simulink model "Channelizer_kernel"  (R2024a)
settings: Solver=VariableStepAuto  StartTime=0.0  StopTime=inf  RelTol=1e-3
InitFcn:
  | init
  | init_kernel
values from neighbouring files (symbols this model uses):
  N = 2*1024    (= 2048)    [hil.m]    (also in init.m = 256)
undefined symbols (not defined in the file or in its folder): ch0, ch1, ch10, ch11, ch12, ch13, ch14, ch15, ch2, ch3, ch4, ch5, ch6, ch7, ch8, ch9, S, vsva2197, xcvc1902
libraries: aieBasic x56, aieUtilities x39, hlsBasic x3, dspindex x2, vmcUtilities x1, commchan3 x1, commrflib2 x1, commfilt2 x1, commrandsrc3 x1, commdigbbndam3 x1
(part 1 of 3)
settings Model: Creator=robg  LastModifiedBy=robg
settings DataIOCC: SaveFormat=Array  SaveOutput=off  SignalLogging=off  DSMLogging=off  SaveTime=off
settings OptimizationCC: ReuseModelBlockBuffer=off
settings DebuggingCC: UnconnectedInputMsg=warning  UnconnectedOutputMsg=warning  UnconnectedLineMsg=warning
settings ModelReferenceCC: EnableRefExpFcnMdlSchedulingChecks=on
settings RTWCC: GPUComputeCapability=3.5  DLArmComputeVersion=19.05

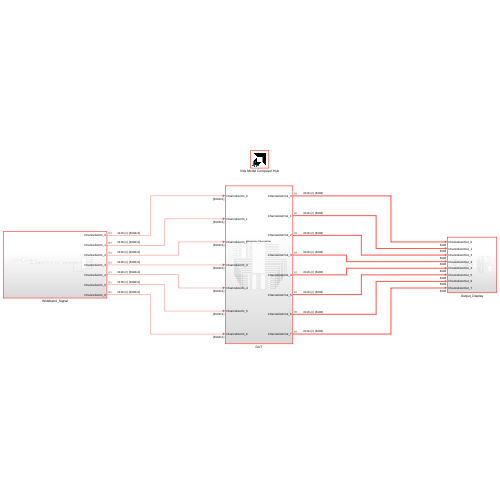
[thumbnail: Simulink's stored preview of the top-level diagram]
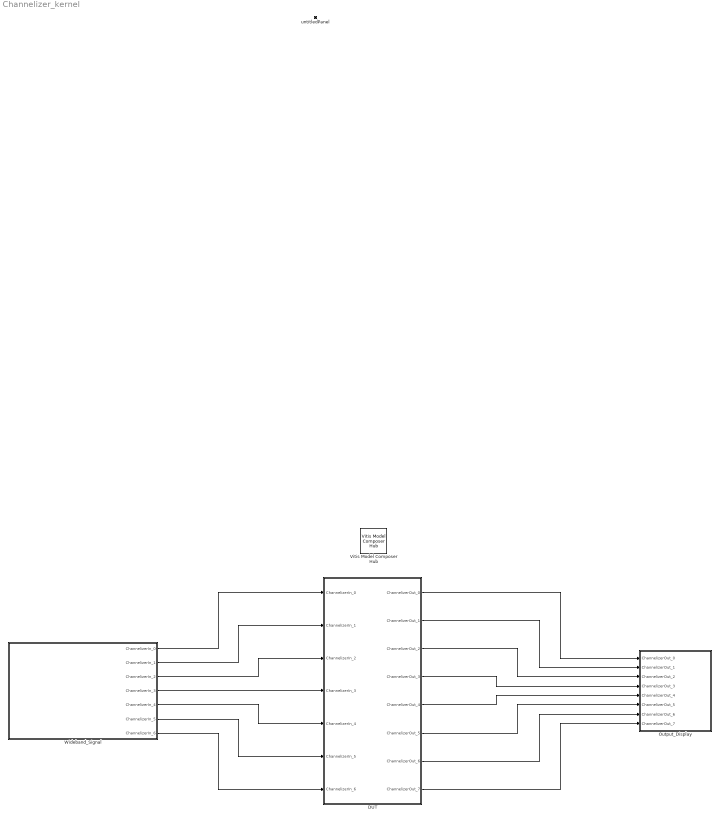
== system Channelizer_kernel ==
  DUT : Subsystem
  Output_Display : Subsystem
  Vitis Model Composer Hub : vmcUtilities/Vitis Model Composer Hub  Tag=genX  CodeGeneration=off  SubsystemName=DUT  DUTSubsystemName=DUT  CompilationType=HWCompilation  SubsystemType=DUTNode  TargetDirectory=./code_hil  exportDesign=off  analyzeDesign=off  validateDesignOnHw=on  ExportType=HW Code  IpVendor=xilinx.com  IpLibrary=hls  IpName=m16_ssr8_permute_fb_o_wrapper  IpVersion=1.0  IpHWLanguage=Verilog  AieCompilerOptions={}  AieSimulatorOptions={}  CreateTestbench=off  TestbenchStackSize=10  RunRtlSim=off  RunCSim=off  RunAieSim=on  AieSimTimeout=50000  RunAieSimProfiling=off  LaunchVitisAnalyzer=off  PlotOutput=off  RunX86Sim=off  X86SimTimeout=10  GenHwImage=off  GenLibadfXo=off  GenHwValidationCode=off  PlatformType=Specify Platform  Platform=/proj/xbuilds/SWIP/2024.1_0306_2227/installs/lin64/Vitis/2024.1/base_platforms/xilinx_vck190_base_202410_1/xilinx_vck190_base_202410_1.xpfm  HwSystemType=Baremetal  HwValidationTarget=hw  ProjDevice=Versal VCK190 Evaluation Platform (xcvc1902-vsva2197-2MP-e-S)  ProjDevicePart=xcvc1902-vsva2197-2MP-e-S  AIEType=AIE  SamplePeriod=-1  ClockFrequency=200  DataPathParallelism=1  xilinxfamily=versalaicore  part=xcvc1902  speed=-2MP-e-S  package=vsva2197  directory=./netlist  testbench=off  incr_netlist=off  synthesis_tool=Vivado  clock_wrapper=Clock Enables  dbl_ovrd=According to Block Masks  dcm_input_clock_period=10  sysclk_period=10  simulink_period=1  eval_field=0  IPInfoJsonString="{\"HLSKernel\":[{\"SubsystemName\":\"m16_ssr8_cyclic_shift_wrapper\",\"IPName\":\"m16_ssr8_cyclic_shift_wrapper\",\"IPLibrary\":\"hls\",\"IPVendor\":\"xilinx.com\",\"IPVersion\":\"1.0\",\"FpgaClockFreq\":\"200\",\"TargetDirectory\":\"./code_hil\",\"SubsystemDir\":\"./code_hil/ip/m16_ssr8_cyclic_shift_wrapper\"},{\"SubsystemName\":\"m16_ssr8_permute_fb_i_wrapper\",\"IPName\":\"m16_ssr8_permute_fb_i_wrapper\",\"IPLibrary\":\"hls\",\"IPVendor\":\"xilinx.com\",\"IPVersion\":\"1.0\",\"FpgaClockFreq\":\"200\",\"TargetDirectory\":\"./code_hil\",\"SubsystemDir\":\"./code_hil/ip/m16_ssr8_permute_fb_i_wrapper\"},{\"SubsystemName\":\"m16_ssr8_permute_fb_o_wrapper\",\"IPName\":\"m16_ssr8_permute_fb_o_wrapper\",\"IPLibrary\":\"hls\",\"IPVendor\":\"xilinx.com\",\"IPVersion\":\"1.0\",\"FpgaClockFreq\":\"200\",\"TargetDirectory\":\"./code_hil\",\"SubsystemDir\":\"./code_hil/ip/m16_ssr8_permute_fb_o_wrapper\"}],\"SubsystemTag\":\"DUTNode\",\"AIESubsystem\":{\"SubsystemName\":\"AIE\",\"TargetDirectory\":\"./code_hil\",\"SubsystemDir\":\"./code_hil/ip/AIE\"}}"  LogFileName=/proj/xsjhdstaff4/abehbood/vmc_examples/gitent/Examples/AIENGINE_plus_PL/AIE_HLS/Channelizer/code_hil/model_composer.log  NThreads=4
  Wideband_Signal : Subsystem
  untitledPanel : Subsystem  Tag=HiddenForWebPanel  IsWebBlockPanel=on
  wires:
  DUT/1(ChannelizerOut_0) -> Output_Display/1(ChannelizerOut_0)
  DUT/2(ChannelizerOut_1) -> Output_Display/2(ChannelizerOut_1)
  DUT/3(ChannelizerOut_2) -> Output_Display/3(ChannelizerOut_2)
  DUT/4(ChannelizerOut_3) -> Output_Display/4(ChannelizerOut_3)
  DUT/5(ChannelizerOut_4) -> Output_Display/5(ChannelizerOut_4)
  DUT/6(ChannelizerOut_5) -> Output_Display/6(ChannelizerOut_5)
  DUT/7(ChannelizerOut_6) -> Output_Display/7(ChannelizerOut_6)
  DUT/8(ChannelizerOut_7) -> Output_Display/8(ChannelizerOut_7)
  Wideband_Signal/4(ChannelizerIn_3) -> DUT/4(ChannelizerIn_3)
  Wideband_Signal/3(ChannelizerIn_2) -> DUT/3(ChannelizerIn_2)
  Wideband_Signal/5(ChannelizerIn_4) -> DUT/5(ChannelizerIn_4)
  Wideband_Signal/6(ChannelizerIn_5) -> DUT/6(ChannelizerIn_5)
  Wideband_Signal/1(ChannelizerIn_0) -> DUT/1(ChannelizerIn_0)
  Wideband_Signal/7(ChannelizerIn_6) -> DUT/7(ChannelizerIn_6)
  Wideband_Signal/2(ChannelizerIn_1) -> DUT/2(ChannelizerIn_1)

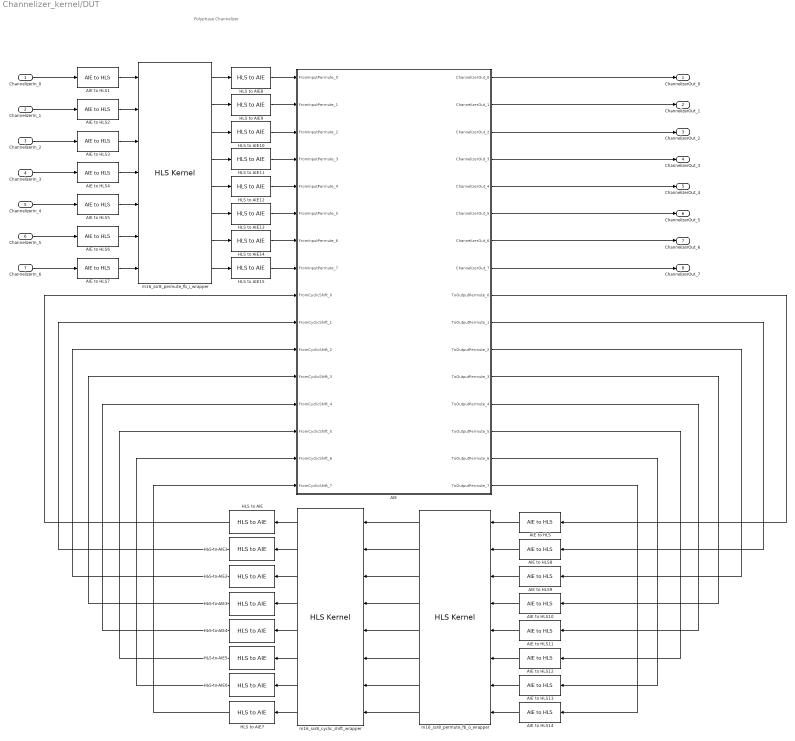
== system Channelizer_kernel/DUT ==
  note: Polyphase Channelizer
  ChannelizerIn_0 : Inport
  ChannelizerIn_1 : Inport  Port=2
  ChannelizerIn_2 : Inport  Port=3
  ChannelizerIn_3 : Inport  Port=4
  ChannelizerIn_4 : Inport  Port=5
  ChannelizerIn_5 : Inport  Port=6
  ChannelizerIn_6 : Inport  Port=7
  AIE : Subsystem
  AIE to HLS{,1..14} (15 alike) : aieUtilities/AIE to HLS  OutputType=ufix128  OutputSize=N
  HLS to AIE{,1..15} (16 alike) : aieUtilities/HLS to AIE  OutputType=cint16  OutputSize=4*N
  m16_ssr8_cyclic_shift_wrapper : hlsBasic/HLS Kernel  PortNames={'return'; 'sig0_i'; 'sig1_i'; 'sig2_i'; 'sig3_i'; 'sig4_i'; 'sig5_i'; 'sig6_i'; 'sig7_i'; 'sig0_o'; 'sig1_o'; 'sig2_o'; 'sig3_o'; 'sig4_o'; 'sig5_o'; 'sig6_o'; 'sig7_o'}  PortSerializedTypes={'{Bv}'; '{R{Thls::stream{2{t{Tap_uint{1{t{}128}}}}{t{}0}}}}'; '{R{Thls::stream{2{t{Tap_uint{1{t{}128}}}}{t{}0}}}}'; '{R{Thls::stream{2{t{Tap_uint{1{t{}128}}}}{t{}0}}}}'; '{R{Thls::stream{2{t{Tap_uint{1{t{}128}}}}{t{}0}}}}'; '{R{Thls::stream{2{t{Tap_uint{1{t{}128}}}}{t{}0}}}}'; '{R{Thls::stream{2{t{Tap_uint{1{t{}128}}}}{t{}0}}}}'; '{R{Thls::stream{2{t{Tap_uint{1{t{}128}}}}{t{}0}}}}'; '{R{Thls::stream{2{t{Tap_uint{1{t{}128}}}}{t{}0}}}}'; '{R{Thls::stream{2{t{Tap_uint{1{t{}128}}}}{t{}0}}}}'; '{R{Thls::stream{2{t{Tap_uint{1{t{}128}}}}{t{}0}}}}'; '{R{Thls::stream{2{t{Tap_uint{1{t{}128}}}}{t{}0}}}}'; '{R{Thls::stream{2{t{Tap_uint{1{t{}128}}}}{t{}0}}}}'; '{R{Thls::stream{2{t{Tap_uint{1{t{}128}}}}{t{}0}}}}'; '{R{Thls::stream{2{t{Tap_uint{1{t{}128}}}}{t{}0}}}}'; '{R{Thls::stream{2{t{Tap_uint{1{t{}128}}}}{t{}0}}}}'; '{R{Thls::stream{2{t{Tap_uint{1{t{}128}}}}{t{}0}}}}'}  FunctionTemplateSpecKind=none  FunctionTemplateParamNames={}  FunctionTemplateParamKinds={}  FunctionTemplateParamTypes={}  FunctionTemplateParamValues={}  PortSynchronicities={'auto'; 'auto'; 'auto'; 'auto'; 'auto'; 'auto'; 'auto'; 'auto'; 'auto'; 'auto'; 'auto'; 'auto'; 'auto'; 'auto'; 'auto'; 'auto'}  PortSignalSizes={0.000000000000000000e+00; 0.000000000000000000e+00; 0.000000000000000000e+00; 0.000000000000000000e+00; 0.000000000000000000e+00; 0.000000000000000000e+00; 0.000000000000000000e+00; 0.000000000000000000e+00; 2.048000000000000000e+03; 2.048000000000000000e+03; 2.048000000000000000e+03; 2.048000000000000000e+03; 2.048000000000000000e+03; 2.048000000000000000e+03; 2.048000000000000000e+03; 2.048000000000000000e+03}  PortParameterValues={}  FunctionTemplateParams={}  FunctionTemplateParamsEnables={}  FunctionTemplateParamsVisible=off  FunctionDeclTypeOptions=C[1 1]@t7@<empty>  PortAttributesTable={ 'Input', 'sig0_i', 'hls::stream< ap_uint< 128 >, 0 > &', '', ''; 'Input', 'sig1_i', 'hls::stream< ap_uint< 128 >, 0 > &', '', ''; 'Input', 'sig2_i', 'hls::stream< ap_uint< 128 >, 0 > &', '', ''; 'Input', 'sig3_i', 'hls::stream< ap_uint< 128 >, 0 > &', '', ''; 'Input', 'sig4_i', 'hls::stream< ap_uint< 128 >, 0 > &', '', ''; 'Input', 'sig5_i', 'hls::stream< ap_uint< 128 >, 0 > &', '', ''; 'Input', 'sig6_i', 'hls::stream< ap_uint< 128 >, 0 > &', '', ''; 'Input', 'sig7_i', 'hls::stream< ap_uint< 128 >, 0 > &', '', ''; 'Output', 'sig0_o', 'hls::stream< ap_uint< 128 >, 0 > &', '', 'N'; 'Output', 'sig1_o', 'hls::stream< ap_uint< 128 >, 0 > &', '', 'N'; 'Output', 'sig2_o', 'hls::stream< ap_uint< 128 >, 0 > &', '', 'N'; 'Output', 'sig3_o', 'hls::stream< ap_uint< 128 >, 0 > &', '', 'N'; 'Output', 'sig4_o', 'hls::stream< ap_uint< 128 >, 0 > &', '', 'N'; 'Output', 'sig5_o', 'hls::stream< ap_uint< 128 >, 0 > &', '', 'N'; 'Output', 'sig6_o', 'hls::stream< ap_uint< 128 >, 0 > &', '', 'N'; 'Output', 'sig7_o', 'hls::stream< ap_uint< 128 >, 0 > &', '', 'N' }  PortAttributesEnablement={'off', 'off', 'off', 'off', 'off';'off', 'off', 'off', 'off', 'off';'off', 'off', 'off', 'off', 'off';'off', 'off', 'off', 'off', 'off';'off', 'off', 'off', 'off', 'off';'off', 'off', 'off', 'off', 'off';'off', 'off', 'off', 'off', 'off';'off', 'off', 'off', 'off', 'off';'off', 'off', 'off', 'off', 'on';'off', 'off', 'off', 'off', 'on';'off', 'off', 'off', 'off', 'on';'off', 'off', 'off', 'off', 'on';'off', 'off', 'off', 'off', 'on';'off', 'off', 'off', 'off', 'on';'off', 'off', 'off', 'off', 'on';'off', 'off', 'off', 'off', 'on'}  PortParametersTable={}  SampleTime=-1  PortDirectionTable={ 'sig0_i', 'hls::stream< ap_uint< 128 >, 0 > &', 'Input', 'Port'; 'sig1_i', 'hls::stream< ap_uint< 128 >, 0 > &', 'Input', 'Port'; 'sig2_i', 'hls::stream< ap_uint< 128 >, 0 > &', 'Input', 'Port'; 'sig3_i', 'hls::stream< ap_uint< 128 >, 0 > &', 'Input', 'Port'; 'sig4_i', 'hls::stream< ap_uint< 128 >, 0 > &', 'Input', 'Port'; 'sig5_i', 'hls::stream< ap_uint< 128 >, 0 > &', 'Input', 'Port'; 'sig6_i', 'hls::stream< ap_uint< 128 >, 0 > &', 'Input', 'Port'; 'sig7_i', 'hls::stream< ap_uint< 128 >, 0 > &', 'Input', 'Port'; 'sig0_o', 'hls::stream< ap_uint< 128 >, 0 > &', 'Output', 'Port'; 'sig1_o', 'hls::stream< ap_uint< 128 >, 0 > &', 'Output', 'Port'; 'sig2_o', 'hls::stream< ap_uint< 128 >, 0 > &', 'Output', 'Port'; 'sig3_o', 'hls::stream< ap_uint< 128 >, 0 > &', 'Output', 'Port'; 'sig4_o', 'hls::stream< ap_uint< 128 >, 0 > &', 'Output', 'Port'; 'sig5_o', 'hls::stream< ap_uint< 128 >, 0 > &', 'Output', 'Port'; 'sig6_o', 'hls::stream< ap_uint< 128 >, 0 > &', 'Output', 'Port'; 'sig7_o', 'hls::stream< ap_uint< 128 >, 0 > &', 'Output', 'Port' }  PortDirectionTabVisible=on  ArgDirections={1.000000000000000000e+00; 1.000000000000000000e+00; 1.000000000000000000e+00; 1.000000000000000000e+00; 1.000000000000000000e+00; 1.000000000000000000e+00; 1.000000000000000000e+00; 1.000000000000000000e+00; 2.000000000000000000e+00; 2.000000000000000000e+00; 2.000000000000000000e+00; 2.000000000000000000e+00; 2.000000000000000000e+00; 2.000000000000000000e+00; 2.000000000000000000e+00; 2.000000000000000000e+00}  ArgInterfaceTypes={1.000000000000000000e+00; 1.000000000000000000e+00; 1.000000000000000000e+00; 1.000000000000000000e+00; 1.000000000000000000e+00; 1.000000000000000000e+00; 1.000000000000000000e+00; 1.000000000000000000e+00; 1.000000000000000000e+00; 1.000000000000000000e+00; 1.000000000000000000e+00; 1.000000000000000000e+00; 1.000000000000000000e+00; 1.000000000000000000e+00; 1.000000000000000000e+00; 1.000000000000000000e+00}  FunctionIndex=1  FormalArgDecls={'hls::stream< ap_uint< 128 >, 0 > & sig0_i', 'hls::stream< ap_uint< 128 >, 0 > & sig1_i', 'hls::stream< ap_uint< 128 >, 0 > & sig2_i', 'hls::stream< ap_uint< 128 >, 0 > & sig3_i', 'hls::stream< ap_uint< 128 >, 0 > & sig4_i', 'hls::stream< ap_uint< 128 >, 0 > & sig5_i', 'hls::stream< ap_uint< 128 >, 0 > & sig6_i', 'hls::stream< ap_uint< 128 >, 0 > & sig7_i', 'hls::stream< ap_uint< 128 >, 0 > & sig0_o', 'hls::stream< ap_uint< 128 >, 0 > & sig1_o', 'hls::stream< ap_uint< 128 >, 0 > & sig2_o', 'hls::stream< ap_uint< 128 >, 0 > & sig3_o', 'hls::stream< ap_uint< 128 >, 0 > & sig4_o', 'hls::stream< ap_uint< 128 >, 0 > & sig5_o', 'hls::stream< ap_uint< 128 >, 0 > & sig6_o', 'hls::stream< ap_uint< 128 >, 0 > & sig7_o'}  SimLibPath=''  FunctionTabVisible=on  FunctionDescription=void m16_ssr8_cyclic_shift_wrapper(hls::stream< ap_uint< 128 >, 0 > & sig0_i, hls::stream< ap_uint< 128 >, 0 > & sig1_i, hls::stream< ap_uint< 128 >, 0 > & sig2_i, hls::stream< ap_uint< 128 >, 0 > & sig3_i, hls::stream< ap_uint< 128 >, 0 > & sig4_i, hls::stream< ap_uint< 128 >, 0 > & sig5_i, hls::stream< ap_uint< 128 >, 0 > & sig6_i, hls::stream< ap_uint< 128 >, 0 > & sig7_i, hls::stream< ap_uint< 128 >, 0 > & sig0_o, hls::stream< ap_uint< 128 >, 0 > & sig1_o, hls::stream< ap_uint< 128 >, 0 > & sig2_o, hls::stream< ap_uint< 128 >, 0 > & sig3_o, hls::stream< ap_uint< 128 >, 0 > & sig4_o, hls::stream< ap_uint< 128 >, 0 > & sig5_o, hls::stream< ap_uint< 128 >, 0 > & sig6_o, hls::stream< ap_uint< 128 >, 0 > & sig7_o)  blockJsonConstraints=[]  deprecateConstraints=0  KernelHeaderFile=hls/m16_ssr8_cyclic_shift.h  KernelFunction=m16_ssr8_cyclic_shift_wrapper  KernelFunctionSelect=<empty>  KernelSourceFile=hls/m16_ssr8_cyclic_shift.cpp  KernelSearchPaths={}  PreProcOptions={}
  m16_ssr8_permute_fb_i_wrapper : hlsBasic/HLS Kernel  PortNames={'return'; 'sig0_i'; 'sig1_i'; 'sig2_i'; 'sig3_i'; 'sig4_i'; 'sig5_i'; 'sig6_i'; 'sig0_o'; 'sig1_o'; 'sig2_o'; 'sig3_o'; 'sig4_o'; 'sig5_o'; 'sig6_o'; 'sig7_o'}  PortSerializedTypes={'{Bv}'; '{R{Thls::stream{2{t{Tap_uint{1{t{}128}}}}{t{}0}}}}'; '{R{Thls::stream{2{t{Tap_uint{1{t{}128}}}}{t{}0}}}}'; '{R{Thls::stream{2{t{Tap_uint{1{t{}128}}}}{t{}0}}}}'; '{R{Thls::stream{2{t{Tap_uint{1{t{}128}}}}{t{}0}}}}'; '{R{Thls::stream{2{t{Tap_uint{1{t{}128}}}}{t{}0}}}}'; '{R{Thls::stream{2{t{Tap_uint{1{t{}128}}}}{t{}0}}}}'; '{R{Thls::stream{2{t{Tap_uint{1{t{}128}}}}{t{}0}}}}'; '{R{Thls::stream{2{t{Tap_uint{1{t{}128}}}}{t{}0}}}}'; '{R{Thls::stream{2{t{Tap_uint{1{t{}128}}}}{t{}0}}}}'; '{R{Thls::stream{2{t{Tap_uint{1{t{}128}}}}{t{}0}}}}'; '{R{Thls::stream{2{t{Tap_uint{1{t{}128}}}}{t{}0}}}}'; '{R{Thls::stream{2{t{Tap_uint{1{t{}128}}}}{t{}0}}}}'; '{R{Thls::stream{2{t{Tap_uint{1{t{}128}}}}{t{}0}}}}'; '{R{Thls::stream{2{t{Tap_uint{1{t{}128}}}}{t{}0}}}}'; '{R{Thls::stream{2{t{Tap_uint{1{t{}128}}}}{t{}0}}}}'}  FunctionTemplateSpecKind=none  FunctionTemplateParamNames={}  FunctionTemplateParamKinds={}  FunctionTemplateParamTypes={}  FunctionTemplateParamValues={}  PortSynchronicities={'auto'; 'auto'; 'auto'; 'auto'; 'auto'; 'auto'; 'auto'; 'auto'; 'auto'; 'auto'; 'auto'; 'auto'; 'auto'; 'auto'; 'auto'}  PortSignalSizes={0.000000000000000000e+00; 0.000000000000000000e+00; 0.000000000000000000e+00; 0.000000000000000000e+00; 0.000000000000000000e+00; 0.000000000000000000e+00; 0.000000000000000000e+00; 2.048000000000000000e+03; 2.048000000000000000e+03; 2.048000000000000000e+03; 2.048000000000000000e+03; 2.048000000000000000e+03; 2.048000000000000000e+03; 2.048000000000000000e+03; 2.048000000000000000e+03}  PortParameterValues={}  FunctionTemplateParams={}  FunctionTemplateParamsEnables={}  FunctionTemplateParamsVisible=off  FunctionDeclTypeOptions=C[1 1]@t7@<empty>  PortAttributesTable={ 'Input', 'sig0_i', 'hls::stream< ap_uint< 128 >, 0 > &', '', ''; 'Input', 'sig1_i', 'hls::stream< ap_uint< 128 >, 0 > &', '', ''; 'Input', 'sig2_i', 'hls::stream< ap_uint< 128 >, 0 > &', '', ''; 'Input', 'sig3_i', 'hls::stream< ap_uint< 128 >, 0 > &', '', ''; 'Input', 'sig4_i', 'hls::stream< ap_uint< 128 >, 0 > &', '', ''; 'Input', 'sig5_i', 'hls::stream< ap_uint< 128 >, 0 > &', '', ''; 'Input', 'sig6_i', 'hls::stream< ap_uint< 128 >, 0 > &', '', ''; 'Output', 'sig0_o', 'hls::stream< ap_uint< 128 >, 0 > &', '', 'N'; 'Output', 'sig1_o', 'hls::stream< ap_uint< 128 >, 0 > &', '', 'N'; 'Output', 'sig2_o', 'hls::stream< ap_uint< 128 >, 0 > &', '', 'N'; 'Output', 'sig3_o', 'hls::stream< ap_uint< 128 >, 0 > &', '', 'N'; 'Output', 'sig4_o', 'hls::stream< ap_uint< 128 >, 0 > &', '', 'N'; 'Output', 'sig5_o', 'hls::stream< ap_uint< 128 >, 0 > &', '', 'N'; 'Output', 'sig6_o', 'hls::stream< ap_uint< 128 >, 0 > &', '', 'N'; 'Output', 'sig7_o', 'hls::stream< ap_uint< 128 >, 0 > &', '', 'N' }  PortAttributesEnablement={'off', 'off', 'off', 'off', 'off';'off', 'off', 'off', 'off', 'off';'off', 'off', 'off', 'off', 'off';'off', 'off', 'off', 'off', 'off';'off', 'off', 'off', 'off', 'off';'off', 'off', 'off', 'off', 'off';'off', 'off', 'off', 'off', 'off';'off', 'off', 'off', 'off', 'on';'off', 'off', 'off', 'off', 'on';'off', 'off', 'off', 'off', 'on';'off', 'off', 'off', 'off', 'on';'off', 'off', 'off', 'off', 'on';'off', 'off', 'off', 'off', 'on';'off', 'off', 'off', 'off', 'on';'off', 'off', 'off', 'off', 'on'}  PortParametersTable={}  SampleTime=-1  PortDirectionTable={ 'sig0_i', 'hls::stream< ap_uint< 128 >, 0 > &', 'Input', 'Port'; 'sig1_i', 'hls::stream< ap_uint< 128 >, 0 > &', 'Input', 'Port'; 'sig2_i', 'hls::stream< ap_uint< 128 >, 0 > &', 'Input', 'Port'; 'sig3_i', 'hls::stream< ap_uint< 128 >, 0 > &', 'Input', 'Port'; 'sig4_i', 'hls::stream< ap_uint< 128 >, 0 > &', 'Input', 'Port'; 'sig5_i', 'hls::stream< ap_uint< 128 >, 0 > &', 'Input', 'Port'; 'sig6_i', 'hls::stream< ap_uint< 128 >, 0 > &', 'Input', 'Port'; 'sig0_o', 'hls::stream< ap_uint< 128 >, 0 > &', 'Output', 'Port'; 'sig1_o', 'hls::stream< ap_uint< 128 >, 0 > &', 'Output', 'Port'; 'sig2_o', 'hls::stream< ap_uint< 128 >, 0 > &', 'Output', 'Port'; 'sig3_o', 'hls::stream< ap_uint< 128 >, 0 > &', 'Output', 'Port'; 'sig4_o', 'hls::stream< ap_uint< 128 >, 0 > &', 'Output', 'Port'; 'sig5_o', 'hls::stream< ap_uint< 128 >, 0 > &', 'Output', 'Port'; 'sig6_o', 'hls::stream< ap_uint< 128 >, 0 > &', 'Output', 'Port'; 'sig7_o', 'hls::stream< ap_uint< 128 >, 0 > &', 'Output', 'Port' }  PortDirectionTabVisible=on  ArgDirections={1.000000000000000000e+00; 1.000000000000000000e+00; 1.000000000000000000e+00; 1.000000000000000000e+00; 1.000000000000000000e+00; 1.000000000000000000e+00; 1.000000000000000000e+00; 2.000000000000000000e+00; 2.000000000000000000e+00; 2.000000000000000000e+00; 2.000000000000000000e+00; 2.000000000000000000e+00; 2.000000000000000000e+00; 2.000000000000000000e+00; 2.000000000000000000e+00}  ArgInterfaceTypes={1.000000000000000000e+00; 1.000000000000000000e+00; 1.000000000000000000e+00; 1.000000000000000000e+00; 1.000000000000000000e+00; 1.000000000000000000e+00; 1.000000000000000000e+00; 1.000000000000000000e+00; 1.000000000000000000e+00; 1.000000000000000000e+00; 1.000000000000000000e+00; 1.000000000000000000e+00; 1.000000000000000000e+00; 1.000000000000000000e+00; 1.000000000000000000e+00}  FunctionIndex=1  FormalArgDecls={'hls::stream< ap_uint< 128 >, 0 > & sig0_i', 'hls::stream< ap_uint< 128 >, 0 > & sig1_i', 'hls::stream< ap_uint< 128 >, 0 > & sig2_i', 'hls::stream< ap_uint< 128 >, 0 > & sig3_i', 'hls::stream< ap_uint< 128 >, 0 > & sig4_i', 'hls::stream< ap_uint< 128 >, 0 > & sig5_i', 'hls::stream< ap_uint< 128 >, 0 > & sig6_i', 'hls::stream< ap_uint< 128 >, 0 > & sig0_o', 'hls::stream< ap_uint< 128 >, 0 > & sig1_o', 'hls::stream< ap_uint< 128 >, 0 > & sig2_o', 'hls::stream< ap_uint< 128 >, 0 > & sig3_o', 'hls::stream< ap_uint< 128 >, 0 > & sig4_o', 'hls::stream< ap_uint< 128 >, 0 > & sig5_o', 'hls::stream< ap_uint< 128 >, 0 > & sig6_o', 'hls::stream< ap_uint< 128 >, 0 > & sig7_o'}  SimLibPath=''  FunctionTabVisible=on  FunctionDescription=void m16_ssr8_permute_fb_i_wrapper(hls::stream< ap_uint< 128 >, 0 > & sig0_i, hls::stream< ap_uint< 128 >, 0 > & sig1_i, hls::stream< ap_uint< 128 >, 0 > & sig2_i, hls::stream< ap_uint< 128 >, 0 > & sig3_i, hls::stream< ap_uint< 128 >, 0 > & sig4_i, hls::stream< ap_uint< 128 >, 0 > & sig5_i, hls::stream< ap_uint< 128 >, 0 > & sig6_i, hls::stream< ap_uint< 128 >, 0 > & sig0_o, hls::stream< ap_uint< 128 >, 0 > & sig1_o, hls::stream< ap_uint< 128 >, 0 > & sig2_o, hls::stream< ap_uint< 128 >, 0 > & sig3_o, hls::stream< ap_uint< 128 >, 0 > & sig4_o, hls::stream< ap_uint< 128 >, 0 > & sig5_o, hls::stream< ap_uint< 128 >, 0 > & sig6_o, hls::stream< ap_uint< 128 >, 0 > & sig7_o)  blockJsonConstraints=[]  deprecateConstraints=0  KernelHeaderFile=hls/m16_ssr8_permute_fb_i.h  KernelFunction=m16_ssr8_permute_fb_i_wrapper  KernelFunctionSelect=<empty>  KernelSourceFile=hls/m16_ssr8_permute_fb_i.cpp  KernelSearchPaths={}  PreProcOptions={}
  m16_ssr8_permute_fb_o_wrapper : hlsBasic/HLS Kernel  PortNames={'return'; 'sig0_i'; 'sig1_i'; 'sig2_i'; 'sig3_i'; 'sig4_i'; 'sig5_i'; 'sig6_i'; 'sig7_i'; 'sig0_o'; 'sig1_o'; 'sig2_o'; 'sig3_o'; 'sig4_o'; 'sig5_o'; 'sig6_o'; 'sig7_o'}  PortSerializedTypes={'{Bv}'; '{R{Thls::stream{2{t{Tap_uint{1{t{}128}}}}{t{}0}}}}'; '{R{Thls::stream{2{t{Tap_uint{1{t{}128}}}}{t{}0}}}}'; '{R{Thls::stream{2{t{Tap_uint{1{t{}128}}}}{t{}0}}}}'; '{R{Thls::stream{2{t{Tap_uint{1{t{}128}}}}{t{}0}}}}'; '{R{Thls::stream{2{t{Tap_uint{1{t{}128}}}}{t{}0}}}}'; '{R{Thls::stream{2{t{Tap_uint{1{t{}128}}}}{t{}0}}}}'; '{R{Thls::stream{2{t{Tap_uint{1{t{}128}}}}{t{}0}}}}'; '{R{Thls::stream{2{t{Tap_uint{1{t{}128}}}}{t{}0}}}}'; '{R{Thls::stream{2{t{Tap_uint{1{t{}128}}}}{t{}0}}}}'; '{R{Thls::stream{2{t{Tap_uint{1{t{}128}}}}{t{}0}}}}'; '{R{Thls::stream{2{t{Tap_uint{1{t{}128}}}}{t{}0}}}}'; '{R{Thls::stream{2{t{Tap_uint{1{t{}128}}}}{t{}0}}}}'; '{R{Thls::stream{2{t{Tap_uint{1{t{}128}}}}{t{}0}}}}'; '{R{Thls::stream{2{t{Tap_uint{1{t{}128}}}}{t{}0}}}}'; '{R{Thls::stream{2{t{Tap_uint{1{t{}128}}}}{t{}0}}}}'; '{R{Thls::stream{2{t{Tap_uint{1{t{}128}}}}{t{}0}}}}'}  FunctionTemplateSpecKind=none  FunctionTemplateParamNames={}  FunctionTemplateParamKinds={}  FunctionTemplateParamTypes={}  FunctionTemplateParamValues={}  PortSynchronicities={'auto'; 'auto'; 'auto'; 'auto'; 'auto'; 'auto'; 'auto'; 'auto'; 'auto'; 'auto'; 'auto'; 'auto'; 'auto'; 'auto'; 'auto'; 'auto'}  PortSignalSizes={0.000000000000000000e+00; 0.000000000000000000e+00; 0.000000000000000000e+00; 0.000000000000000000e+00; 0.000000000000000000e+00; 0.000000000000000000e+00; 0.000000000000000000e+00; 0.000000000000000000e+00; 2.048000000000000000e+03; 2.048000000000000000e+03; 2.048000000000000000e+03; 2.048000000000000000e+03; 2.048000000000000000e+03; 2.048000000000000000e+03; 2.048000000000000000e+03; 2.048000000000000000e+03}  PortParameterValues={}  FunctionTemplateParams={}  FunctionTemplateParamsEnables={}  FunctionTemplateParamsVisible=off  FunctionDeclTypeOptions=C[1 1]@t7@<empty>  PortAttributesTable={ 'Input', 'sig0_i', 'hls::stream< ap_uint< 128 >, 0 > &', '', ''; 'Input', 'sig1_i', 'hls::stream< ap_uint< 128 >, 0 > &', '', ''; 'Input', 'sig2_i', 'hls::stream< ap_uint< 128 >, 0 > &', '', ''; 'Input', 'sig3_i', 'hls::stream< ap_uint< 128 >, 0 > &', '', ''; 'Input', 'sig4_i', 'hls::stream< ap_uint< 128 >, 0 > &', '', ''; 'Input', 'sig5_i', 'hls::stream< ap_uint< 128 >, 0 > &', '', ''; 'Input', 'sig6_i', 'hls::stream< ap_uint< 128 >, 0 > &', '', ''; 'Input', 'sig7_i', 'hls::stream< ap_uint< 128 >, 0 > &', '', ''; 'Output', 'sig0_o', 'hls::stream< ap_uint< 128 >, 0 > &', '', 'N'; 'Output', 'sig1_o', 'hls::stream< ap_uint< 128 >, 0 > &', '', 'N'; 'Output', 'sig2_o', 'hls::stream< ap_uint< 128 >, 0 > &', '', 'N'; 'Output', 'sig3_o', 'hls::stream< ap_uint< 128 >, 0 > &', '', 'N'; 'Output', 'sig4_o', 'hls::stream< ap_uint< 128 >, 0 > &', '', 'N'; 'Output', 'sig5_o', 'hls::stream< ap_uint< 128 >, 0 > &', '', 'N'; 'Output', 'sig6_o', 'hls::stream< ap_uint< 128 >, 0 > &', '', 'N'; 'Output', 'sig7_o', 'hls::stream< ap_uint< 128 >, 0 > &', '', 'N' }  PortAttributesEnablement={'off', 'off', 'off', 'off', 'off';'off', 'off', 'off', 'off', 'off';'off', 'off', 'off', 'off', 'off';'off', 'off', 'off', 'off', 'off';'off', 'off', 'off', 'off', 'off';'off', 'off', 'off', 'off', 'off';'off', 'off', 'off', 'off', 'off';'off', 'off', 'off', 'off', 'off';'off', 'off', 'off', 'off', 'on';'off', 'off', 'off', 'off', 'on';'off', 'off', 'off', 'off', 'on';'off', 'off', 'off', 'off', 'on';'off', 'off', 'off', 'off', 'on';'off', 'off', 'off', 'off', 'on';'off', 'off', 'off', 'off', 'on';'off', 'off', 'off', 'off', 'on'}  PortParametersTable={}  SampleTime=-1  PortDirectionTable={ 'sig0_i', 'hls::stream< ap_uint< 128 >, 0 > &', 'Input', 'Port'; 'sig1_i', 'hls::stream< ap_uint< 128 >, 0 > &', 'Input', 'Port'; 'sig2_i', 'hls::stream< ap_uint< 128 >, 0 > &', 'Input', 'Port'; 'sig3_i', 'hls::stream< ap_uint< 128 >, 0 > &', 'Input', 'Port'; 'sig4_i', 'hls::stream< ap_uint< 128 >, 0 > &', 'Input', 'Port'; 'sig5_i', 'hls::stream< ap_uint< 128 >, 0 > &', 'Input', 'Port'; 'sig6_i', 'hls::stream< ap_uint< 128 >, 0 > &', 'Input', 'Port'; 'sig7_i', 'hls::stream< ap_uint< 128 >, 0 > &', 'Input', 'Port'; 'sig0_o', 'hls::stream< ap_uint< 128 >, 0 > &', 'Output', 'Port'; 'sig1_o', 'hls::stream< ap_uint< 128 >, 0 > &', 'Output', 'Port'; 'sig2_o', 'hls::stream< ap_uint< 128 >, 0 > &', 'Output', 'Port'; 'sig3_o', 'hls::stream< ap_uint< 128 >, 0 > &', 'Output', 'Port'; 'sig4_o', 'hls::stream< ap_uint< 128 >, 0 > &', 'Output', 'Port'; 'sig5_o', 'hls::stream< ap_uint< 128 >, 0 > &', 'Output', 'Port'; 'sig6_o', 'hls::stream< ap_uint< 128 >, 0 > &', 'Output', 'Port'; 'sig7_o', 'hls::stream< ap_uint< 128 >, 0 > &', 'Output', 'Port' }  PortDirectionTabVisible=on  ArgDirections={1.000000000000000000e+00; 1.000000000000000000e+00; 1.000000000000000000e+00; 1.000000000000000000e+00; 1.000000000000000000e+00; 1.000000000000000000e+00; 1.000000000000000000e+00; 1.000000000000000000e+00; 2.000000000000000000e+00; 2.000000000000000000e+00; 2.000000000000000000e+00; 2.000000000000000000e+00; 2.000000000000000000e+00; 2.000000000000000000e+00; 2.000000000000000000e+00; 2.000000000000000000e+00}  ArgInterfaceTypes={1.000000000000000000e+00; 1.000000000000000000e+00; 1.000000000000000000e+00; 1.000000000000000000e+00; 1.000000000000000000e+00; 1.000000000000000000e+00; 1.000000000000000000e+00; 1.000000000000000000e+00; 1.000000000000000000e+00; 1.000000000000000000e+00; 1.000000000000000000e+00; 1.000000000000000000e+00; 1.000000000000000000e+00; 1.000000000000000000e+00; 1.000000000000000000e+00; 1.000000000000000000e+00}  FunctionIndex=1  FormalArgDecls={'hls::stream< ap_uint< 128 >, 0 > & sig0_i', 'hls::stream< ap_uint< 128 >, 0 > & sig1_i', 'hls::stream< ap_uint< 128 >, 0 > & sig2_i', 'hls::stream< ap_uint< 128 >, 0 > & sig3_i', 'hls::stream< ap_uint< 128 >, 0 > & sig4_i', 'hls::stream< ap_uint< 128 >, 0 > & sig5_i', 'hls::stream< ap_uint< 128 >, 0 > & sig6_i', 'hls::stream< ap_uint< 128 >, 0 > & sig7_i', 'hls::stream< ap_uint< 128 >, 0 > & sig0_o', 'hls::stream< ap_uint< 128 >, 0 > & sig1_o', 'hls::stream< ap_uint< 128 >, 0 > & sig2_o', 'hls::stream< ap_uint< 128 >, 0 > & sig3_o', 'hls::stream< ap_uint< 128 >, 0 > & sig4_o', 'hls::stream< ap_uint< 128 >, 0 > & sig5_o', 'hls::stream< ap_uint< 128 >, 0 > & sig6_o', 'hls::stream< ap_uint< 128 >, 0 > & sig7_o'}  SimLibPath=''  FunctionTabVisible=on  FunctionDescription=void m16_ssr8_permute_fb_o_wrapper(hls::stream< ap_uint< 128 >, 0 > & sig0_i, hls::stream< ap_uint< 128 >, 0 > & sig1_i, hls::stream< ap_uint< 128 >, 0 > & sig2_i, hls::stream< ap_uint< 128 >, 0 > & sig3_i, hls::stream< ap_uint< 128 >, 0 > & sig4_i, hls::stream< ap_uint< 128 >, 0 > & sig5_i, hls::stream< ap_uint< 128 >, 0 > & sig6_i, hls::stream< ap_uint< 128 >, 0 > & sig7_i, hls::stream< ap_uint< 128 >, 0 > & sig0_o, hls::stream< ap_uint< 128 >, 0 > & sig1_o, hls::stream< ap_uint< 128 >, 0 > & sig2_o, hls::stream< ap_uint< 128 >, 0 > & sig3_o, hls::stream< ap_uint< 128 >, 0 > & sig4_o, hls::stream< ap_uint< 128 >, 0 > & sig5_o, hls::stream< ap_uint< 128 >, 0 > & sig6_o, hls::stream< ap_uint< 128 >, 0 > & sig7_o)  blockJsonConstraints=[]  deprecateConstraints=0  KernelHeaderFile=hls/m16_ssr8_permute_fb_o.h  KernelFunction=m16_ssr8_permute_fb_o_wrapper  KernelFunctionSelect=<empty>  KernelSourceFile=hls/m16_ssr8_permute_fb_o.cpp  KernelSearchPaths={}  PreProcOptions={}
  ChannelizerOut_0 : Outport
  ChannelizerOut_1 : Outport  Port=2
  ChannelizerOut_2 : Outport  Port=3
  ChannelizerOut_3 : Outport  Port=4
  ChannelizerOut_4 : Outport  Port=5
  ChannelizerOut_5 : Outport  Port=6
  ChannelizerOut_6 : Outport  Port=7
  ChannelizerOut_7 : Outport  Port=8
  wires:
  m16_ssr8_cyclic_shift_wrapper/1 -> HLS to AIE/1
  m16_ssr8_cyclic_shift_wrapper/8 -> HLS to AIE7/1
  m16_ssr8_cyclic_shift_wrapper/6 -> HLS to AIE5/1
  m16_ssr8_cyclic_shift_wrapper/4 -> HLS to AIE3/1
  m16_ssr8_cyclic_shift_wrapper/7 -> HLS to AIE6/1
  m16_ssr8_cyclic_shift_wrapper/3 -> HLS to AIE2/1
  m16_ssr8_cyclic_shift_wrapper/2 -> HLS to AIE1/1
  m16_ssr8_cyclic_shift_wrapper/5 -> HLS to AIE4/1
  AIE/9(ToOutputPermute_0) -> AIE to HLS/1
  AIE/10(ToOutputPermute_1) -> AIE to HLS8/1
  AIE/11(ToOutputPermute_2) -> AIE to HLS9/1
  AIE/12(ToOutputPermute_3) -> AIE to HLS10/1
  AIE/13(ToOutputPermute_4) -> AIE to HLS11/1
  AIE/14(ToOutputPermute_5) -> AIE to HLS12/1
  AIE/15(ToOutputPermute_6) -> AIE to HLS13/1
  AIE/16(ToOutputPermute_7) -> AIE to HLS14/1
  HLS to AIE/1 -> AIE/9(FromCyclicShift_0)
  HLS to AIE1/1 -> AIE/10(FromCyclicShift_1)
  HLS to AIE2/1 -> AIE/11(FromCyclicShift_2)
  HLS to AIE3/1 -> AIE/12(FromCyclicShift_3)
  HLS to AIE4/1 -> AIE/13(FromCyclicShift_4)
  HLS to AIE5/1 -> AIE/14(FromCyclicShift_5)
  HLS to AIE6/1 -> AIE/15(FromCyclicShift_6)
  HLS to AIE7/1 -> AIE/16(FromCyclicShift_7)
  AIE/5(ChannelizerOut_4) -> ChannelizerOut_4/1
  AIE/6(ChannelizerOut_5) -> ChannelizerOut_5/1
  AIE/7(ChannelizerOut_6) -> ChannelizerOut_6/1
  AIE/8(ChannelizerOut_7) -> ChannelizerOut_7/1
  AIE/4(ChannelizerOut_3) -> ChannelizerOut_3/1
  AIE/3(ChannelizerOut_2) -> ChannelizerOut_2/1
  AIE/2(ChannelizerOut_1) -> ChannelizerOut_1/1
  AIE/1(ChannelizerOut_0) -> ChannelizerOut_0/1
  AIE to HLS4/1 -> m16_ssr8_permute_fb_i_wrapper/4
  AIE to HLS7/1 -> m16_ssr8_permute_fb_i_wrapper/7
  m16_ssr8_permute_fb_i_wrapper/6 -> HLS to AIE13/1
  AIE to HLS1/1 -> m16_ssr8_permute_fb_i_wrapper/1
  AIE to HLS2/1 -> m16_ssr8_permute_fb_i_wrapper/2
  m16_ssr8_permute_fb_i_wrapper/7 -> HLS to AIE14/1
  AIE to HLS3/1 -> m16_ssr8_permute_fb_i_wrapper/3
  m16_ssr8_permute_fb_i_wrapper/8 -> HLS to AIE15/1
  m16_ssr8_permute_fb_i_wrapper/5 -> HLS to AIE12/1
  AIE to HLS6/1 -> m16_ssr8_permute_fb_i_wrapper/6
  m16_ssr8_permute_fb_i_wrapper/3 -> HLS to AIE10/1
  m16_ssr8_permute_fb_i_wrapper/1 -> HLS to AIE8/1
  m16_ssr8_permute_fb_i_wrapper/4 -> HLS to AIE11/1
  AIE to HLS5/1 -> m16_ssr8_permute_fb_i_wrapper/5
  m16_ssr8_permute_fb_i_wrapper/2 -> HLS to AIE9/1
  AIE to HLS/1 -> m16_ssr8_permute_fb_o_wrapper/1
  AIE to HLS8/1 -> m16_ssr8_permute_fb_o_wrapper/2
  AIE to HLS9/1 -> m16_ssr8_permute_fb_o_wrapper/3
  AIE to HLS10/1 -> m16_ssr8_permute_fb_o_wrapper/4
  AIE to HLS11/1 -> m16_ssr8_permute_fb_o_wrapper/5
  AIE to HLS12/1 -> m16_ssr8_permute_fb_o_wrapper/6
  AIE to HLS13/1 -> m16_ssr8_permute_fb_o_wrapper/7
  AIE to HLS14/1 -> m16_ssr8_permute_fb_o_wrapper/8
  m16_ssr8_permute_fb_o_wrapper/1 -> m16_ssr8_cyclic_shift_wrapper/1
  m16_ssr8_permute_fb_o_wrapper/2 -> m16_ssr8_cyclic_shift_wrapper/2
  m16_ssr8_permute_fb_o_wrapper/3 -> m16_ssr8_cyclic_shift_wrapper/3
  m16_ssr8_permute_fb_o_wrapper/4 -> m16_ssr8_cyclic_shift_wrapper/4
  m16_ssr8_permute_fb_o_wrapper/5 -> m16_ssr8_cyclic_shift_wrapper/5
  m16_ssr8_permute_fb_o_wrapper/6 -> m16_ssr8_cyclic_shift_wrapper/6
  m16_ssr8_permute_fb_o_wrapper/7 -> m16_ssr8_cyclic_shift_wrapper/7
  m16_ssr8_permute_fb_o_wrapper/8 -> m16_ssr8_cyclic_shift_wrapper/8
  ChannelizerIn_0/1 -> AIE to HLS1/1
  ChannelizerIn_1/1 -> AIE to HLS2/1
  ChannelizerIn_2/1 -> AIE to HLS3/1
  ChannelizerIn_3/1 -> AIE to HLS4/1
  ChannelizerIn_4/1 -> AIE to HLS5/1
  ChannelizerIn_5/1 -> AIE to HLS6/1
  ChannelizerIn_6/1 -> AIE to HLS7/1
  HLS to AIE8/1 -> AIE/1(FromInputPermute_0)
  HLS to AIE9/1 -> AIE/2(FromInputPermute_1)
  HLS to AIE10/1 -> AIE/3(FromInputPermute_2)
  HLS to AIE11/1 -> AIE/4(FromInputPermute_3)
  HLS to AIE12/1 -> AIE/5(FromInputPermute_4)
  HLS to AIE13/1 -> AIE/6(FromInputPermute_5)
  HLS to AIE14/1 -> AIE/7(FromInputPermute_6)
  HLS to AIE15/1 -> AIE/8(FromInputPermute_7)

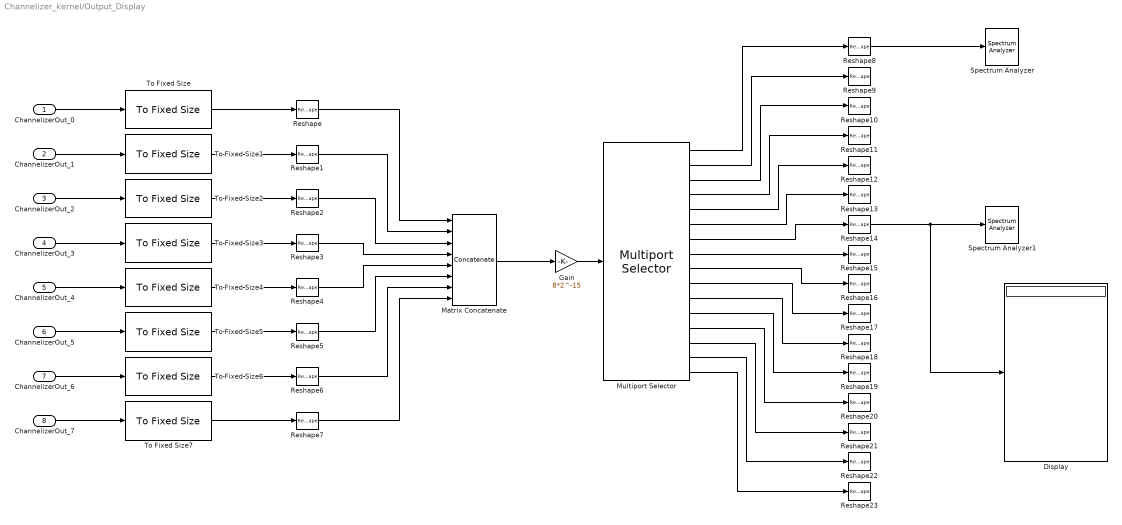
== system Channelizer_kernel/Output_Display ==
  ChannelizerOut_0 : Inport
  ChannelizerOut_1 : Inport  Port=2
  ChannelizerOut_2 : Inport  Port=3
  ChannelizerOut_3 : Inport  Port=4
  ChannelizerOut_4 : Inport  Port=5
  ChannelizerOut_5 : Inport  Port=6
  ChannelizerOut_6 : Inport  Port=7
  ChannelizerOut_7 : Inport  Port=8
  Display : Display
  Gain : Gain  Gain=8*2^-15  OutDataTypeStr=double
  Matrix Concatenate : Concatenate  NumInputs=8  Mode=Multidimensional array
  Multiport Selector : dspindex/Multiport Selector  rowsOrCols=Rows  idxCellArray={[1,5], [2,6], [3,7],[4,8],[9,13],[10,14],[11,15],[12,16],[17,21],[18,22],[19 23],[20 24],[25 29],[26 30],[27 31],[28 32]}  idxErrMode=Generate Error
      settings: LibrarySourceBlock=|
      | dsphdlsupportsigmgmt/Multiport
      | Selector
  Reshape{,1..7} (8 alike) : Reshape  OutputDimensionality=Customize  OutputDimensions=[4,N]
  Reshape{8..23} (16 alike) : Reshape
  Spectrum Analyzer : SpectrumAnalyzer  WindowPosition=[1957.000000,239.000000,383.000000,383.000000,]  Visible=on  ScopeFrameLocation=window  AxesScaling=Manual  Span=625000000  StartFrequency=-312500000  StopFrequency=312500000  Title=Channel 0  YLimits=[-50,10]
  Spectrum Analyzer1 : SpectrumAnalyzer  WindowPosition=[1948.000000,668.000000,383.000000,383.000000,]  Visible=on  ScopeFrameLocation=window  AxesScaling=Manual  Span=625000000  StartFrequency=-312500000  StopFrequency=312500000  Title=Channel 6  YLimits=[-50,10]
  To Fixed Size{,1..7} (8 alike) : aieUtilities/To Fixed Size  Mode=Stop simulation when input variable-size signal is not full  OutputSize=Inherit: Same as input  CopyMethod=Buffer samples to form output  HasStatusOutput=on
  wires:
  ChannelizerOut_7/1 -> To Fixed Size7/1
  ChannelizerOut_4/1 -> To Fixed Size4/1
  ChannelizerOut_2/1 -> To Fixed Size2/1
  ChannelizerOut_5/1 -> To Fixed Size5/1
  ChannelizerOut_3/1 -> To Fixed Size3/1
  ChannelizerOut_1/1 -> To Fixed Size1/1
  To Fixed Size6/1 -> Reshape6/1
  To Fixed Size3/1 -> Reshape3/1
  To Fixed Size4/1 -> Reshape4/1
  To Fixed Size2/1 -> Reshape2/1
  To Fixed Size/1 -> Reshape/1
  To Fixed Size5/1 -> Reshape5/1
  To Fixed Size1/1 -> Reshape1/1
  ChannelizerOut_0/1 -> To Fixed Size/1
  To Fixed Size7/1 -> Reshape7/1
  ChannelizerOut_6/1 -> To Fixed Size6/1
  Reshape/1 -> Matrix Concatenate/1
  Reshape1/1 -> Matrix Concatenate/2
  Reshape4/1 -> Matrix Concatenate/5
  Reshape3/1 -> Matrix Concatenate/4
  Reshape5/1 -> Matrix Concatenate/6
  Reshape2/1 -> Matrix Concatenate/3
  Reshape6/1 -> Matrix Concatenate/7
  Reshape7/1 -> Matrix Concatenate/8
  Matrix Concatenate/1 -> Gain/1
  Multiport Selector/1 -> Reshape8/1
  Multiport Selector/2 -> Reshape9/1
  Multiport Selector/3 -> Reshape10/1
  Multiport Selector/4 -> Reshape11/1
  Multiport Selector/5 -> Reshape12/1
  Multiport Selector/6 -> Reshape13/1
  Multiport Selector/7 -> Reshape14/1
  Multiport Selector/8 -> Reshape15/1
  Multiport Selector/9 -> Reshape16/1
  Multiport Selector/10 -> Reshape17/1
  Multiport Selector/11 -> Reshape18/1
  Multiport Selector/12 -> Reshape19/1
  Multiport Selector/13 -> Reshape20/1
  Multiport Selector/14 -> Reshape21/1
  Multiport Selector/15 -> Reshape22/1
  Multiport Selector/16 -> Reshape23/1
  Reshape8/1 -> Spectrum Analyzer/1
  Gain/1 -> Multiport Selector/1
  Reshape14/1 -> Display/1, Spectrum Analyzer1/1

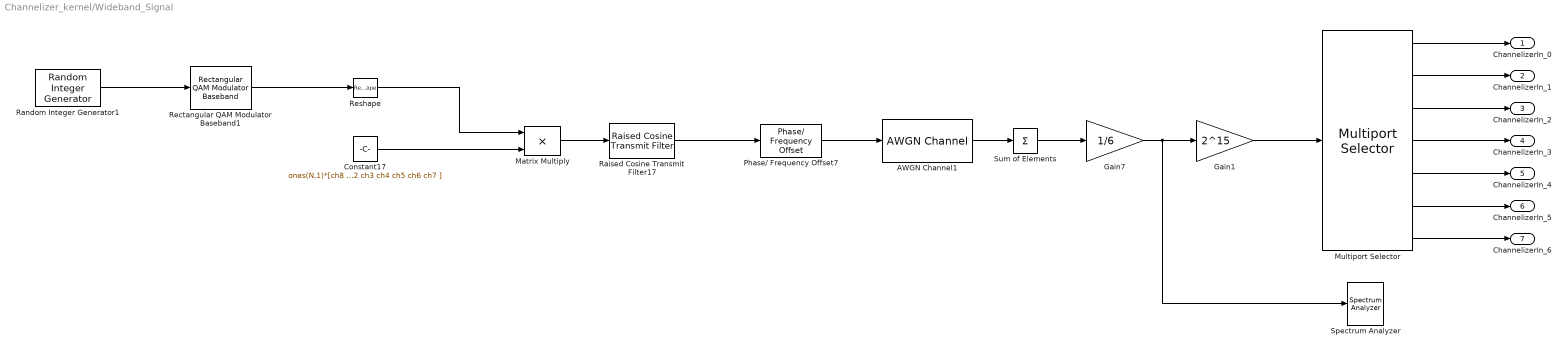
== system Channelizer_kernel/Wideband_Signal ==
  AWGN Channel1 : commchan3/AWGN Channel  LegacyMode=on  NoiseMethod="Signal to noise ratio  (SNR)"  noiseMode="Signal to noise ratio  (SNR)"  EbNo=10  EsNo=10  SNR=10  BitsPerSymbol=1  SignalPower=1  SamplesPerSymbol=1  SymbolPeriod=1  VarianceSource=Parameter  Variance=1  RandomStream=Global stream  Seed=67  SimulateUsing=Code generation
  Constant17 : Constant  Value=ones(N,1)*[ch8 ch9 ch10 ch11 ch12 ch13 ch14 ch15 ch0 ch1 ch2 ch3 ch4 ch5 ch6 ch7 ]  SampleTime=-1
  Gain1 : Gain  Gain=2^15  OutDataTypeStr=int16
  Gain7 : Gain  Gain=1/6  OutDataTypeStr=double
  Matrix Multiply : Product
  Multiport Selector : dspindex/Multiport Selector  rowsOrCols=Rows  idxCellArray={I1, I2, I3, I4, I5, I6, I7}  idxErrMode=Clip Index
  Phase/ Frequency Offset7 : commrflib2/Phase// Frequency Offset  phaseOffset=0  freqPort=off  freqOffset="[-8  -7 -6 -5 -4 -3 -2 -1 0 1 2 3 4 5 6 7]*8.75e9 / 16"
  Raised Cosine Transmit Filter17 : commfilt2/Raised Cosine Transmit Filter  filtType=Normal  R=0.3  filtSpan=10  N=28  filterGain=1  InputProcessing=Columns as channels (frame based)  RateOptions=Enforce single-rate processing  framing=Mute  checkCoeff=off  variableName=rcTxFilt17  checkGain=Normalized  sampMode=Mute  saveAsFlag=0  currentFiltSpan=10  D=(10)/2  launchFVT=on  roundingMode=Floor  overflowMode=off  coeffDataTypeStr=Inherit: Same word length as input  coeffMin=[]  coeffMax=[]  coeffLastDataTypeStr=Inherit: Same word length as input  outputDataTypeStr=Inherit: Same as accumulator  outputMin=[]  outputMax=[]  outputLastDataTypeStr=Inherit: Same as accumulator
  Random Integer Generator1 : commrandsrc3/Random Integer Generator  SetSize=16  SeedSource=Auto  Seed=0  SampleTime=(7/4)/8.75e9  SamplesPerFrame=16*N  OutputDataType=double  SimulateUsing=Interpreted execution
  Rectangular QAM Modulator Baseband1 : commdigbbndam3/Rectangular QAM Modulator Baseband  M=16  InType=Integer  Enc=Gray  Mapping=[0:15]  PowType=Min. distance between symbols  MinDist=2  AvgPow=1  PeakPow=1  Ph=0  outDtype=double  outWordLen=16  outUDDataType=sfix(16)  outFracLenMode=Best precision  outFracLen=15  outDataTypeStr=double  outLastDataTypeStr=double
  Reshape : Reshape  OutputDimensionality=Customize  OutputDimensions=[N,16]
  Spectrum Analyzer : SpectrumAnalyzer  WindowPosition=[740.000000,171.000000,800.000000,500.000000,]  Visible=on  ScopeFrameLocation=window  SpectrumType=Power density  ViewType=Spectrum and spectrogram  Span=8750000000  StartFrequency=-4375000000  StopFrequency=4375000000  AveragingMethod=Exponential  SpectrumUnits=dBm/Hz  YLimits=[-88.21338427,-70.38302075]  ColorLimits=[-88.21338427,-70.38302075]  AllowFFTLengthLessThanSamplesPerUpdate=on
  Sum of Elements : Sum  Inputs=+  CollapseMode=Specified dimension  CollapseDim=2
  ChannelizerIn_0 : Outport
  ChannelizerIn_1 : Outport  Port=2
  ChannelizerIn_2 : Outport  Port=3
  ChannelizerIn_3 : Outport  Port=4
  ChannelizerIn_4 : Outport  Port=5
  ChannelizerIn_5 : Outport  Port=6
  ChannelizerIn_6 : Outport  Port=7
  wires:
  Multiport Selector/1 -> ChannelizerIn_0/1
  Rectangular QAM Modulator Baseband1/1 -> Reshape/1
  AWGN Channel1/1 -> Sum of Elements/1
  Multiport Selector/7 -> ChannelizerIn_6/1
  Raised Cosine Transmit Filter17/1 -> Phase/ Frequency Offset7/1
  Random Integer Generator1/1 -> Rectangular QAM Modulator Baseband1/1
  Constant17/1 -> Matrix Multiply/2
  Multiport Selector/3 -> ChannelizerIn_2/1
  Multiport Selector/4 -> ChannelizerIn_3/1
  Matrix Multiply/1 -> Raised Cosine Transmit Filter17/1
  Multiport Selector/6 -> ChannelizerIn_5/1
  Multiport Selector/5 -> ChannelizerIn_4/1
  Multiport Selector/2 -> ChannelizerIn_1/1
  Reshape/1 -> Matrix Multiply/1
  Sum of Elements/1 -> Gain7/1
  Gain7/1 -> Spectrum Analyzer/1, Gain1/1
  Phase/ Frequency Offset7/1 -> AWGN Channel1/1
  Gain1/1 -> Multiport Selector/1

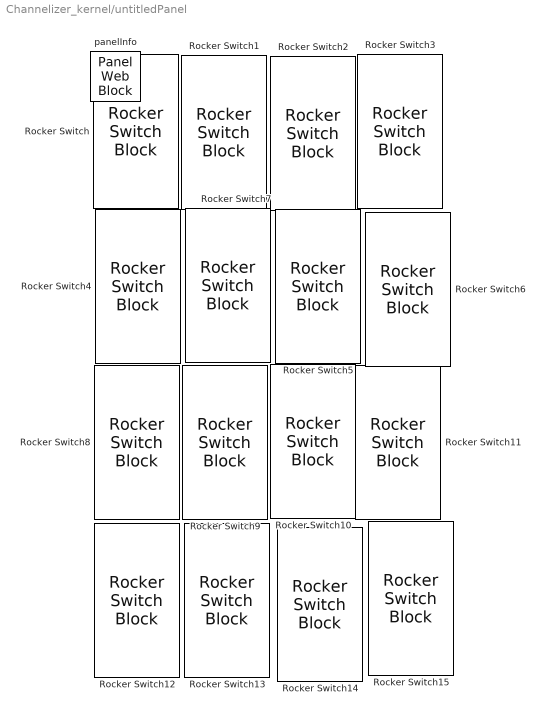
== system Channelizer_kernel/untitledPanel ==
  Rocker Switch : RockerSwitchBlock  Tag=HiddenForWebPanel  PanelInfo="{\"height\":154,\"left\":10,\"panelId\":\"panelId-fec1c322-f5e7-4e4f-8c31-b98d6132c1cd\",\"top\":12,\"type\":\"panelChild\",\"version\":\"2019b\",\"width\":85,\"zIndex\":1500002}"
      settings: Values={{'Off', 'On'}, [0 1]}
  Rocker Switch1 : RockerSwitchBlock  Tag=HiddenForWebPanel  PanelInfo="{\"height\":154,\"left\":98,\"panelId\":\"panelId-fec1c322-f5e7-4e4f-8c31-b98d6132c1cd\",\"top\":12,\"type\":\"panelChild\",\"version\":\"2019b\",\"width\":85,\"zIndex\":1500004}"
      settings: Values={{'Off', 'On'}, [0 1]}
  Rocker Switch10 : RockerSwitchBlock  Tag=HiddenForWebPanel  PanelInfo="{\"height\":154,\"left\":185,\"panelId\":\"panelId-fec1c322-f5e7-4e4f-8c31-b98d6132c1cd\",\"top\":327,\"type\":\"panelChild\",\"version\":\"2019b\",\"width\":85,\"zIndex\":1500022}"
      settings: Values={{'Off', 'On'}, [0 1]}
  Rocker Switch11 : RockerSwitchBlock  Tag=HiddenForWebPanel  PanelInfo="{\"height\":154,\"left\":273,\"panelId\":\"panelId-fec1c322-f5e7-4e4f-8c31-b98d6132c1cd\",\"top\":327,\"type\":\"panelChild\",\"version\":\"2019b\",\"width\":85,\"zIndex\":1500024}"
      settings: Values={{'Off', 'On'}, [0 1]}
  Rocker Switch12 : RockerSwitchBlock  Tag=HiddenForWebPanel  PanelInfo="{\"height\":154,\"left\":10,\"panelId\":\"panelId-fec1c322-f5e7-4e4f-8c31-b98d6132c1cd\",\"top\":483,\"type\":\"panelChild\",\"version\":\"2019b\",\"width\":85,\"zIndex\":1500026}"
      settings: Values={{'Off', 'On'}, [0 1]}
  Rocker Switch13 : RockerSwitchBlock  Tag=HiddenForWebPanel  PanelInfo="{\"height\":154,\"left\":97,\"panelId\":\"panelId-fec1c322-f5e7-4e4f-8c31-b98d6132c1cd\",\"top\":483,\"type\":\"panelChild\",\"version\":\"2019b\",\"width\":85,\"zIndex\":1500028}"
      settings: Values={{'Off', 'On'}, [0 1]}
  Rocker Switch14 : RockerSwitchBlock  Tag=HiddenForWebPanel  PanelInfo="{\"height\":154,\"left\":185,\"panelId\":\"panelId-fec1c322-f5e7-4e4f-8c31-b98d6132c1cd\",\"top\":484,\"type\":\"panelChild\",\"version\":\"2019b\",\"width\":85,\"zIndex\":1500030}"
      settings: Values={{'Off', 'On'}, [0 1]}
  Rocker Switch15 : RockerSwitchBlock  Tag=HiddenForWebPanel  PanelInfo="{\"height\":154,\"left\":272,\"panelId\":\"panelId-fec1c322-f5e7-4e4f-8c31-b98d6132c1cd\",\"top\":484,\"type\":\"panelChild\",\"version\":\"2019b\",\"width\":85,\"zIndex\":1500032}"
      settings: Values={{'Off', 'On'}, [0 1]}
  Rocker Switch2 : RockerSwitchBlock  Tag=HiddenForWebPanel  PanelInfo="{\"height\":154,\"left\":186,\"panelId\":\"panelId-fec1c322-f5e7-4e4f-8c31-b98d6132c1cd\",\"top\":12,\"type\":\"panelChild\",\"version\":\"2019b\",\"width\":85,\"zIndex\":1500006}"
      settings: Values={{'Off', 'On'}, [0 1]}
  Rocker Switch3 : RockerSwitchBlock  Tag=HiddenForWebPanel  PanelInfo="{\"height\":154,\"left\":274,\"panelId\":\"panelId-fec1c322-f5e7-4e4f-8c31-b98d6132c1cd\",\"top\":12,\"type\":\"panelChild\",\"version\":\"2019b\",\"width\":85,\"zIndex\":1500008}"
      settings: Values={{'Off', 'On'}, [0 1]}
  Rocker Switch4 : RockerSwitchBlock  Tag=HiddenForWebPanel  PanelInfo="{\"height\":154,\"left\":10,\"panelId\":\"panelId-fec1c322-f5e7-4e4f-8c31-b98d6132c1cd\",\"top\":169,\"type\":\"panelChild\",\"version\":\"2019b\",\"width\":85,\"zIndex\":1500010}"
      settings: Values={{'Off', 'On'}, [0 1]}
  Rocker Switch5 : RockerSwitchBlock  Tag=HiddenForWebPanel  PanelInfo="{\"height\":154,\"left\":186,\"panelId\":\"panelId-fec1c322-f5e7-4e4f-8c31-b98d6132c1cd\",\"top\":170,\"type\":\"panelChild\",\"version\":\"2019b\",\"width\":85,\"zIndex\":1500012}"
      settings: Values={{'Off', 'On'}, [0 1]}
  Rocker Switch6 : RockerSwitchBlock  Tag=HiddenForWebPanel  PanelInfo="{\"height\":154,\"left\":274,\"panelId\":\"panelId-fec1c322-f5e7-4e4f-8c31-b98d6132c1cd\",\"top\":170,\"type\":\"panelChild\",\"version\":\"2019b\",\"width\":85,\"zIndex\":1500014}"
      settings: Values={{'Off', 'On'}, [0 1]}
  Rocker Switch7 : RockerSwitchBlock  Tag=HiddenForWebPanel  PanelInfo="{\"height\":154,\"left\":98,\"panelId\":\"panelId-fec1c322-f5e7-4e4f-8c31-b98d6132c1cd\",\"top\":169,\"type\":\"panelChild\",\"version\":\"2019b\",\"width\":85,\"zIndex\":1500016}"
      settings: Values={{'Off', 'On'}, [0 1]}
  Rocker Switch8 : RockerSwitchBlock  Tag=HiddenForWebPanel  PanelInfo="{\"height\":154,\"left\":10,\"panelId\":\"panelId-fec1c322-f5e7-4e4f-8c31-b98d6132c1cd\",\"top\":326,\"type\":\"panelChild\",\"version\":\"2019b\",\"width\":85,\"zIndex\":1500018}"
      settings: Values={{'Off', 'On'}, [0 1]}
  Rocker Switch9 : RockerSwitchBlock  Tag=HiddenForWebPanel  PanelInfo="{\"height\":154,\"left\":97,\"panelId\":\"panelId-fec1c322-f5e7-4e4f-8c31-b98d6132c1cd\",\"top\":326,\"type\":\"panelChild\",\"version\":\"2019b\",\"width\":85,\"zIndex\":1500020}"
      settings: Values={{'Off', 'On'}, [0 1]}
  panelInfo : PanelWebBlock  Tag=HiddenForWebPanel  PanelInfo="{\"compacted\":false,\"height\":655,\"isActiveTab\":true,\"left\":-4,\"name\":\"Panel\",\"panelId\":\"panelId-fec1c322-f5e7-4e4f-8c31-b98d6132c1cd\",\"tabIndex\":0,\"tabbedSetId\":\"tabbedSet6868322055\",\"top\":96,\"type\":\"panel\",\"version\":\"2019b\",\"visible\":true,\"width\":371,\"zIndex\":1500002}"  PanelSnapshot=<binary blob, 10492 chars, not shown>
